simulink model "HyperscaleDataCenter"  (R2025b)
settings: Solver=VariableStepAuto  StartTime=0.0  StopTime=10  FixedStep=5e-5  RelTol=1e-4
PostLoadFcn:
  | HyperscaleDataCenterParam
values from neighbouring files (symbols this model uses):
  baseVoltageDC = 800    [DataCenterBBUParam.m]    (also in HyperscaleDataCenterParam.m; UPSBESSParam.m)
  bess_Ki = bess.controller.Ki    [SSTBESSParam.m]
  bess_Kp = bess.controller.Kp    [SSTBESSParam.m]
  droopGain = 0.02    [HyperscaleDataCenterParam.m]    (also in SSTBESSParam.m; UPSBESSParam.m)
  peakShavingPowerLimit = 800e3    (= 800000)    [HyperscaleDataCenterParam.m]
  powerTau = 0.005    [HyperscaleDataCenterParam.m]
  Prated_batt = 40e3    (= 40000)    [HyperscaleDataCenterParam.m]
  tauPS = 0.1    [HyperscaleDataCenterParam.m]
  Ts = 50e-6    (= 5e-05)    [BBUParam.m]    (also in DataCenterBBUParam.m; HyperscaleDataCenterParam.m)
  Ts_PS = 1e-3    (= 0.001)    [HyperscaleDataCenterParam.m]
undefined symbols (not defined in the file or in its folder): bbu, DiscIntNeverNeededParam, dspblkCoreblockFVToolHelper, ee_sli_rtmsupport, gcbh, grid, rack, sst, ups
libraries: fl_lib x80, nesl_utility x42, datacenter_lib x20, ee_lib x17, simulink x10, eeGeneralControl x9, slpidlib x6, microgridRenewables_lib x4, eeTransforms x4, batteryecm_lib x3, eeSinusoidalMeasurementV2 x2, simulink_extras x1
(part 3 of 5)

== system HyperscaleDataCenter/Server Load/Racks/Inference Rack ==
  U_in : Inport
  FaultFlag : Inport  Port=2
  Capacitor : fl_lib/Electrical/Electrical Elements/Capacitor  c=20e-3 F  r=1e-6 Ohm  g=0 1/Ohm  i_specify=off  i_priority=None  i=0 A  i_nominal_specify=off  i_nominal_value=1  i_nominal_unit=A  v_specify=off  v_priority=None  v=0 V  v_nominal_specify=off  v_nominal_value=1  v_nominal_unit=V  vc_specify=on  vc_priority=None  vc=800 V  vc_nominal_specify=off  vc_nominal_value=1  vc_nominal_unit=V
  Current Sensor : fl_lib/Electrical/Electrical Sensors/Current Sensor
  Dynamic Load : ee_lib/Passive/Dynamic Load  load_type=ee.enum.dc_ac.dc  min_supply_voltage=20 V  pow_min=1e-3 W  G_reverse=1e-6 S  deltaV=1e-3 V  f0=60 Hz  Vrms_min=200 V  tau=0.001 s  Vrms_ini=300 V  Vang_ini=0 deg
      settings: InternalSimscapePortConfiguration="{\"Bottom\":[],\"Left\":[{\"id\":\"p\",\"label\":\"+\",\"type\":\"foundation.electrical.electrical\"}],\"Right\":[{\"id\":\"n\",\"label\":\"-\",\"type\":\"foundation.electrical.electrical\"}],\"Top\":[{\"id\":\"P\",\"label\":\"P\",\"type\":\"input\"}]}"
  Efficiency Gain : fl_lib/Physical Signals/Functions/PS Gain  gain=rack.efficiencyGain
  Hybrid BBU : Subsystem  mask{includeSupercap=on, ctrl_Ts=Ts, ctrl_Vdc_ref=baseVoltageDC, scap_deadZone=bbu.scap.deadZone, scap_Kp=bbu.scap.Kp, scap_Imax=bbu.scap.Imax, scap_capacitance=bbu.scap.capacitance, scap_ESR=bbu.scap.ESR, scap_lpfAlpha=bbu.scap.lpfAlpha, batt_deadZone=bbu.batt.deadZone, batt_Imax=bbu.batt.Imax, batt_Vnom=bbu.batt.Vnom, batt_R1=bbu.batt.R1, batt_lpfAlpha=bbu.batt.lpfAlpha, batt_Kp_ctrl=bbu.batt.Kp_ctrl, batt_Ki_ctrl=bbu.batt.Ki_ctrl}
      mask prompts: includeSupercap "Include Supercapacitor"; ctrl_Ts "Controller sample time"; ctrl_Vdc_ref "DC bus voltage reference"; scap_deadZone "Dead Zone (V)"; scap_Kp "Droop Gain (A/V)"; scap_Imax "Current Limit (A)"; scap_capacitance "Capacitance (F)"; scap_ESR "ESR (Ohm)"; scap_lpfAlpha "SuperCap LPF alpha"; batt_deadZone "Dead Zone (V)"; batt_Imax "Current Limit (A)"; batt_Vnom "Nominal Voltage (V)"; batt_R1 "Internal Resistance (Ohm)"; batt_lpfAlpha "Battery LPF alpha"; batt_Kp_ctrl "Battery PI Kp"; batt_Ki_ctrl "Battery PI Ki"
      mask help: Hybrid Battery Backup Unit with frequency-separated supercapacitor (ms-range) and battery (sec-range) control.
      mask init:
      | % BBU Mask Initialization
      | 
      | % Handle supercapacitor inclusion
      | scPath = [gcb, '/Super Capacitor'];
      | if includeSupercap
      |     set_param(scPath, 'Commented', 'off');
      |     set_param([scPath, '/Droop Gate'], 'LowerValue', num2str(-scap_deadZone), 'UpperValue', num2str(scap_deadZone));
      |     set_param([scPath, '/Kp'], 'Gain', num2str(scap_Kp));
      |     set_param([scPath, '/Iref Sat'], 'UpperLimit', '0', 'LowerLimit', num2str(-scap_Imax));
      |     set_param([scPath, '/Capacitor'], 'c', num2str(scap_capacitance), 'r', num2str(scap_ESR));
      |     set_param([scPath, '/LPF'], 'Numerator', ['[' num2str(1-scap_lpfAlpha) ']'], 'Denominator', ['[1 ' num2str(-scap_lpfAlpha) ']']);
      | else
      |     set_param(scPath, 'Commented', 'on');
      | end
      | 
      | % Propagate battery parameters
      | btPath = [gcb, '/Battery'];
      | set_param([btPath, '/Droop Gate'], 'LowerValue', num2str(-batt_deadZone), 'UpperValue', num2str(batt_deadZone));
      | set_param([btPath, '/Iref Sat'], 'UpperLimit', '0', 'LowerLimit', num2str(-batt_Imax));
      | set_param([btPath, '/Battery'], 'Vnom', num2str(batt_Vnom), 'R1', num2str(batt_R1));
      | set_param([btPath, '/LPF'], 'Numerator', ['[' num2str(1-batt_lpfAlpha) ']'], 'Denominator', ['[1 ' num2str(-batt_lpfAlpha) ']']);
      mask Callback includeSupercap:
      | maskObj = Simulink.Mask.get(gcb);
      | scapEnabled = strcmp(get_param(gcb, 'includeSupercap'), 'on');
      | scapParams = {'scap_deadZone','scap_Kp','scap_Imax','scap_filterTau','scap_capacitance','scap_ESR'};
      | for i = 1:numel(scapParams)
      |     p = maskObj.getParameter(scapParams{i});
      |     if scapEnabled
      |         p.Visible = 'on';
      |     else
      |         p.Visible = 'off';
      |     end
      | end
      mask DialogControl ConfigTab Prompt: Configuration
      mask DialogControl SupercapTab Prompt: Supercapacitor
      mask DialogControl BatteryTab Prompt: Battery
      mask Display: image('hybrid_bbu_icon.png');
  PDU Racks : Subsystem  mask{nTrays=rack.nTrays, nRacks=rack.nRacks, trayMass=rack.trayMass, trayCp=rack.trayCp, trayThermalR=rack.trayThermalR, nGPU=rack.nGPU, gpuTDPperDie=rack.gpuTDPperDie, gpuIdlePower=rack.gpuIdlePower, gpuHBMpower=rack.gpuHBMpower, gpuExponent=rack.gpuExponent, gpuHBMutil=rack.gpuHBMutil, gpuLeakage=rack.gpuLeakage, gpuNominalDieT=rack.gpuNominalDieT, gpuDieThermalC=rack.gpuDieThermalC, gpuHeatSinkR=rack.gpuHeatSinkR, gpuSurfArea=rack.gpuSurfArea, gpuAmbientR=rack.gpuAmbientR, nCPU=rack.nCPU, cpuTDPperSocket=rack.cpuTDPperSocket, cpuIdlePower=rack.cpuIdlePower, cpuExponent=rack.cpuExponent, cpuLeakage=rack.cpuLeakage, cpuNominalDieT=rack.cpuNominalDieT, cpuDieThermalC=rack.cpuDieThermalC, cpuHeatSinkR=rack.cpuHeatSinkR, cpuSurfArea=rack.cpuSurfArea, cpuAmbientR=rack.cpuAmbientR, initialT=rack.initialT, htc=rack.htc}
      mask prompts: nTrays "Number of IT trays per rack (-)"; nRacks "Number of racks (-)"; trayMass "Tray mass (kg)"; trayCp "Tray specific heat capacity (J/kg*K)"; trayThermalR "Tray to external thermal resistance (K/W)"; nGPU "Number of GPU per tray (-)"; gpuTDPperDie "GPU TDP per die (W)"; gpuIdlePower "GPU idle power (W)"; gpuHBMpower "HBM power per GPU (W)"; gpuExponent "GPU power utilization exponent (-)"; gpuHBMutil "HBM utilization as fraction of compute utilization (-)"; gpuLeakage "Leakage increase per K above nominal temperature (W/K)"; gpuNominalDieT "Nominal die temperature at TDP (K)"; gpuDieThermalC "GPU die thermal capacitance (J/K)"; gpuHeatSinkR "GPU die-heat-sink thermal resistance (K/W)"; gpuSurfArea "Surface area per die for ambient heat transfer (m^2)"; gpuAmbientR "GPU die-ambient thermal resistance (K/W)"; nCPU "Number of CPU per tray (-)"; cpuTDPperSocket "CPU TDP per socket (W)"; cpuIdlePower "CPU idle power per socket (W)"; cpuExponent "CPU power utilization exponent (-)"; cpuLeakage "Leakage increase per K above nominal temperature (W/K)"; cpuNominalDieT "Nominal die temperature at TDP (K)"; cpuDieThermalC "CPU die thermal capacitance (J/K)"; cpuHeatSinkR "CPU die-heat-sink thermal resistance (K/W)"; cpuSurfArea "Surface area per die for ambient heat transfer (m^2)"; cpuAmbientR "CPU die-ambient thermal resistance (K/W)"; initialT "Initial temperature (K)"; htc "Heat transfer coefficient to ambient (W/m^2.K)"
      settings: CopyFcn=set_param(gcbh,'LinkStatus','none');  PortSchema="{\"entries\":[{\"content\":{\"sides\":[{\"content\":{\"connectorIds\":[\"LConn1\",\"LConn2\",\"LConn3\"]},\"type\":\"ConnectorPlacement.EquallySpacedRectSide\",\"uuid\":\"1a9a884a-dab1-4495-bf62-c6b2de6c1039\"},{\"content\":{\"connectorIds\":[\"RConn1\",\"RConn2\",\"RConn3\"],\"side\":\"RIGHT\"},\"type\":\"ConnectorPlacement.EquallySpacedRectSide\",\"uuid\":\"05c53434-51c1-4fee-b885-c321dcda8b6b\"},{\"content\":{\"side\":\"TOP\"},\"type\":\"ConnectorPlacement.EquallySpacedRectSide\",\"uuid\":\"c7b5c534-d596-4858-a133-27f005e6c9d4\"},{\"content\":{\"connectorIds\":[\"RConn4\"],\"side\":\"BOTTOM\"},\"type\":\"ConnectorPlacement.EquallySpacedRectSide\",\"uuid\":\"693f3c99-4296-4d86-bfcc-da753d3e576f\"}]},\"type\":\"ConnectorPlacement.EquallySpacedConnector\",\"uuid\":\"ed91c467-c4d0-403f-af16-bac0257594fd\"}],\"packageUris\":[\"http://schema.mathworks.com/mf0/Connector/R2020b\"],\"version\":\"1.0\"}"
      mask Help: web("DocumentationPDURacks.html")
      mask DialogControl Container10 Prompt: PDU Racks
      mask DialogControl getRatingButton Prompt: Get Rating
      mask DialogControl Container9 Prompt: IT Tray
      mask DialogControl Container6 Prompt: GPU
      mask DialogControl Container7 Prompt: CPU
      mask DialogControl Container8 Prompt: Initial Conditions
      mask Display: image('icon_PDURacks.png');
  PS-Simulink Converter1 : nesl_utility/PS-Simulink Converter  PhysicalDomain=network_engine_domain  SubClassName=ps_output  LeftPortType=input  RightPortType=output  PseudoPeriodic=off  Frequencies=[]  VectorFormat=inherit  Unit=inherit  AffineConversion=off
  PS-Simulink Converter2 : nesl_utility/PS-Simulink Converter  PhysicalDomain=network_engine_domain  SubClassName=ps_output  LeftPortType=input  RightPortType=output  PseudoPeriodic=off  Frequencies=[]  VectorFormat=inherit  Unit=inherit  AffineConversion=off
  Product : Product
  SP Conv U : nesl_utility/Simulink-PS Converter  PhysicalDomain=network_engine_domain  SubClassName=ps_input  LeftPortType=input  RightPortType=output  PseudoPeriodic=off  Frequencies=[]  NoiseDistribution=none  NoiseParameters=[]  Unit=1  AffineConversion=off  FilteringAndDerivatives=provide  SimscapeFilterOrder=1  InputFilterTimeConstant=0.001  UdotUserProvided=0
  TermC_Ha : fl_lib/Thermal/Thermal Elements/Thermal Mass  mass_type=foundation.enum.constant_variable.constant  mass=1e4 kg  sp_heat=1000 J/(K*kg)  mass_min=1e-6 kg  num_ports=foundation.enum.numPorts2.one  m_specify=off  m_priority=None  m=1 kg  m_nominal_specify=off  m_nominal_value=1  m_nominal_unit=kg  T_specify=off  T_priority=None  T=308.15 K  T_nominal_specify=off  T_nominal_value=1  T_nominal_unit=K  Q_specify=off  Q_priority=None  Q=0 W  Q_nominal_specify=off  Q_nominal_value=1  Q_nominal_unit=W
  TermC_Hc : fl_lib/Thermal/Thermal Elements/Thermal Mass  mass_type=foundation.enum.constant_variable.constant  mass=1e4 kg  sp_heat=1000 J/(K*kg)  mass_min=1e-6 kg  num_ports=foundation.enum.numPorts2.one  m_specify=off  m_priority=None  m=1 kg  m_nominal_specify=off  m_nominal_value=1  m_nominal_unit=kg  T_specify=off  T_priority=None  T=308.15 K  T_nominal_specify=off  T_nominal_value=1  T_nominal_unit=K  Q_specify=off  Q_priority=None  Q=0 W  Q_nominal_specify=off  Q_nominal_value=1  Q_nominal_unit=W
  Terminator : Terminator
  Voltage Sensor : fl_lib/Electrical/Electrical Sensors/Voltage Sensor
  + : PMIOPort  Side=Left
  - : PMIOPort  Port=2  Side=Left
  wires:
  PS-Simulink Converter2/1 -> Product/2, Hybrid BBU/1(Vdc_meas)  "Vdc_train"
  U_in/1 -> SP Conv U/1
  FaultFlag/1 -> Hybrid BBU/2(FaultFlag)
  PS-Simulink Converter1/1 -> Product/1
  Product/1 -> Terminator/1
  connections:
  PS-Simulink Converter2/LConn1 -- Voltage Sensor/RConn1
  Voltage Sensor/RConn2 -- Hybrid BBU/LConn2 -- Dynamic Load/RConn1 -- -/RConn1 -- Capacitor/RConn1
  SP Conv U/RConn1 -- PDU Racks/LConn2 -- PDU Racks/LConn1
  Capacitor/LConn1 -- Current Sensor/RConn2 -- Dynamic Load/LConn1
  PS-Simulink Converter1/LConn1 -- Current Sensor/RConn1
  Efficiency Gain/RConn1 -- Dynamic Load/LConn2
  Hybrid BBU/LConn1 -- +/RConn1 -- Current Sensor/LConn1 -- Voltage Sensor/LConn1
  PDU Racks/RConn1 -- Efficiency Gain/LConn1
  PDU Racks/LConn3 -- TermC_Ha/LConn1
  PDU Racks/RConn4 -- TermC_Hc/LConn1

== system HyperscaleDataCenter/Server Load/Racks/Training Rack ==
  U_in : Inport
  FaultFlag : Inport  Port=2
  Capacitor : fl_lib/Electrical/Electrical Elements/Capacitor  c=20e-3 F  r=1e-6 Ohm  g=0 1/Ohm  i_specify=off  i_priority=None  i=0 A  i_nominal_specify=off  i_nominal_value=1  i_nominal_unit=A  v_specify=off  v_priority=None  v=0 V  v_nominal_specify=off  v_nominal_value=1  v_nominal_unit=V  vc_specify=on  vc_priority=None  vc=800 V  vc_nominal_specify=off  vc_nominal_value=1  vc_nominal_unit=V
  Current Sensor : fl_lib/Electrical/Electrical Sensors/Current Sensor
  Dynamic Load : ee_lib/Passive/Dynamic Load  load_type=ee.enum.dc_ac.dc  min_supply_voltage=20 V  pow_min=1e-3 W  G_reverse=1e-6 S  deltaV=1e-3 V  f0=60 Hz  Vrms_min=200 V  tau=0.001 s  Vrms_ini=300 V  Vang_ini=0 deg
      settings: InternalSimscapePortConfiguration="{\"Bottom\":[],\"Left\":[{\"id\":\"p\",\"label\":\"+\",\"type\":\"foundation.electrical.electrical\"}],\"Right\":[{\"id\":\"n\",\"label\":\"-\",\"type\":\"foundation.electrical.electrical\"}],\"Top\":[{\"id\":\"P\",\"label\":\"P\",\"type\":\"input\"}]}"
  Efficiency Gain : fl_lib/Physical Signals/Functions/PS Gain  gain=rack.efficiencyGain
  Hybrid BBU : Subsystem  mask{includeSupercap=on, ctrl_Ts=Ts, ctrl_Vdc_ref=baseVoltageDC, scap_deadZone=bbu.scap.deadZone, scap_Kp=bbu.scap.Kp, scap_Imax=bbu.scap.Imax, scap_capacitance=bbu.scap.capacitance, scap_ESR=bbu.scap.ESR, scap_lpfAlpha=bbu.scap.lpfAlpha, batt_deadZone=bbu.batt.deadZone, batt_Imax=bbu.batt.Imax, batt_Vnom=bbu.batt.Vnom, batt_R1=bbu.batt.R1, batt_lpfAlpha=bbu.batt.lpfAlpha, batt_Kp_ctrl=bbu.batt.Kp_ctrl, batt_Ki_ctrl=bbu.batt.Ki_ctrl}
      mask prompts: includeSupercap "Include Supercapacitor"; ctrl_Ts "Controller sample time"; ctrl_Vdc_ref "DC bus voltage reference"; scap_deadZone "Dead Zone (V)"; scap_Kp "Droop Gain (A/V)"; scap_Imax "Current Limit (A)"; scap_capacitance "Capacitance (F)"; scap_ESR "ESR (Ohm)"; scap_lpfAlpha "SuperCap LPF alpha"; batt_deadZone "Dead Zone (V)"; batt_Imax "Current Limit (A)"; batt_Vnom "Nominal Voltage (V)"; batt_R1 "Internal Resistance (Ohm)"; batt_lpfAlpha "Battery LPF alpha"; batt_Kp_ctrl "Battery PI Kp"; batt_Ki_ctrl "Battery PI Ki"
      mask help: Hybrid Battery Backup Unit with frequency-separated supercapacitor (ms-range) and battery (sec-range) control.
      mask init: same as HyperscaleDataCenter/Server Load/Racks/Inference Rack/Hybrid BBU
      mask Callback includeSupercap:
      | maskObj = Simulink.Mask.get(gcb);
      | scapEnabled = strcmp(get_param(gcb, 'includeSupercap'), 'on');
      | scapParams = {'scap_deadZone','scap_Kp','scap_Imax','scap_filterTau','scap_capacitance','scap_ESR'};
      | for i = 1:numel(scapParams)
      |     p = maskObj.getParameter(scapParams{i});
      |     if scapEnabled
      |         p.Visible = 'on';
      |     else
      |         p.Visible = 'off';
      |     end
      | end
      mask DialogControl ConfigTab Prompt: Configuration
      mask DialogControl SupercapTab Prompt: Supercapacitor
      mask DialogControl BatteryTab Prompt: Battery
      mask Display: image('hybrid_bbu_icon.png');
  PDU Racks : Subsystem  mask{nTrays=rack.nTrays, nRacks=rack.nRacks, trayMass=rack.trayMass, trayCp=rack.trayCp, trayThermalR=rack.trayThermalR, nGPU=rack.nGPU, gpuTDPperDie=rack.gpuTDPperDie, gpuIdlePower=rack.gpuIdlePower, gpuHBMpower=rack.gpuHBMpower, gpuExponent=rack.gpuExponent, gpuHBMutil=rack.gpuHBMutil, gpuLeakage=rack.gpuLeakage, gpuNominalDieT=rack.gpuNominalDieT, gpuDieThermalC=rack.gpuDieThermalC, gpuHeatSinkR=rack.gpuHeatSinkR, gpuSurfArea=rack.gpuSurfArea, gpuAmbientR=rack.gpuAmbientR, nCPU=rack.nCPU, cpuTDPperSocket=rack.cpuTDPperSocket, cpuIdlePower=rack.cpuIdlePower, cpuExponent=rack.cpuExponent, cpuLeakage=rack.cpuLeakage, cpuNominalDieT=rack.cpuNominalDieT, cpuDieThermalC=rack.cpuDieThermalC, cpuHeatSinkR=rack.cpuHeatSinkR, cpuSurfArea=rack.cpuSurfArea, cpuAmbientR=rack.cpuAmbientR, initialT=rack.initialT, htc=rack.htc}
      mask prompts: nTrays "Number of IT trays per rack (-)"; nRacks "Number of racks (-)"; trayMass "Tray mass (kg)"; trayCp "Tray specific heat capacity (J/kg*K)"; trayThermalR "Tray to external thermal resistance (K/W)"; nGPU "Number of GPU per tray (-)"; gpuTDPperDie "GPU TDP per die (W)"; gpuIdlePower "GPU idle power (W)"; gpuHBMpower "HBM power per GPU (W)"; gpuExponent "GPU power utilization exponent (-)"; gpuHBMutil "HBM utilization as fraction of compute utilization (-)"; gpuLeakage "Leakage increase per K above nominal temperature (W/K)"; gpuNominalDieT "Nominal die temperature at TDP (K)"; gpuDieThermalC "GPU die thermal capacitance (J/K)"; gpuHeatSinkR "GPU die-heat-sink thermal resistance (K/W)"; gpuSurfArea "Surface area per die for ambient heat transfer (m^2)"; gpuAmbientR "GPU die-ambient thermal resistance (K/W)"; nCPU "Number of CPU per tray (-)"; cpuTDPperSocket "CPU TDP per socket (W)"; cpuIdlePower "CPU idle power per socket (W)"; cpuExponent "CPU power utilization exponent (-)"; cpuLeakage "Leakage increase per K above nominal temperature (W/K)"; cpuNominalDieT "Nominal die temperature at TDP (K)"; cpuDieThermalC "CPU die thermal capacitance (J/K)"; cpuHeatSinkR "CPU die-heat-sink thermal resistance (K/W)"; cpuSurfArea "Surface area per die for ambient heat transfer (m^2)"; cpuAmbientR "CPU die-ambient thermal resistance (K/W)"; initialT "Initial temperature (K)"; htc "Heat transfer coefficient to ambient (W/m^2.K)"
      settings: CopyFcn=set_param(gcbh,'LinkStatus','none');  PortSchema="{\"entries\":[{\"content\":{\"sides\":[{\"content\":{\"connectorIds\":[\"LConn1\",\"LConn2\",\"LConn3\"]},\"type\":\"ConnectorPlacement.EquallySpacedRectSide\",\"uuid\":\"1a9a884a-dab1-4495-bf62-c6b2de6c1039\"},{\"content\":{\"connectorIds\":[\"RConn1\",\"RConn2\",\"RConn3\"],\"side\":\"RIGHT\"},\"type\":\"ConnectorPlacement.EquallySpacedRectSide\",\"uuid\":\"05c53434-51c1-4fee-b885-c321dcda8b6b\"},{\"content\":{\"side\":\"TOP\"},\"type\":\"ConnectorPlacement.EquallySpacedRectSide\",\"uuid\":\"c7b5c534-d596-4858-a133-27f005e6c9d4\"},{\"content\":{\"connectorIds\":[\"RConn4\"],\"side\":\"BOTTOM\"},\"type\":\"ConnectorPlacement.EquallySpacedRectSide\",\"uuid\":\"693f3c99-4296-4d86-bfcc-da753d3e576f\"}]},\"type\":\"ConnectorPlacement.EquallySpacedConnector\",\"uuid\":\"ed91c467-c4d0-403f-af16-bac0257594fd\"}],\"packageUris\":[\"http://schema.mathworks.com/mf0/Connector/R2020b\"],\"version\":\"1.0\"}"
      mask Help: web("DocumentationPDURacks.html")
      mask DialogControl Container10 Prompt: PDU Racks
      mask DialogControl getRatingButton Prompt: Get Rating
      mask DialogControl Container9 Prompt: IT Tray
      mask DialogControl Container6 Prompt: GPU
      mask DialogControl Container7 Prompt: CPU
      mask DialogControl Container8 Prompt: Initial Conditions
      mask Display: image('icon_PDURacks.png');
  PS-Simulink Converter : nesl_utility/PS-Simulink Converter  PhysicalDomain=network_engine_domain  SubClassName=ps_output  LeftPortType=input  RightPortType=output  PseudoPeriodic=off  Frequencies=[]  VectorFormat=inherit  Unit=inherit  AffineConversion=off
  PS-Simulink Converter1 : nesl_utility/PS-Simulink Converter  PhysicalDomain=network_engine_domain  SubClassName=ps_output  LeftPortType=input  RightPortType=output  PseudoPeriodic=off  Frequencies=[]  VectorFormat=inherit  Unit=inherit  AffineConversion=off
  PS-Simulink Converter2 : nesl_utility/PS-Simulink Converter  PhysicalDomain=network_engine_domain  SubClassName=ps_output  LeftPortType=input  RightPortType=output  PseudoPeriodic=off  Frequencies=[]  VectorFormat=inherit  Unit=inherit  AffineConversion=off
  Product : Product
  SP Conv U : nesl_utility/Simulink-PS Converter  PhysicalDomain=network_engine_domain  SubClassName=ps_input  LeftPortType=input  RightPortType=output  PseudoPeriodic=off  Frequencies=[]  NoiseDistribution=none  NoiseParameters=[]  Unit=1  AffineConversion=off  FilteringAndDerivatives=provide  SimscapeFilterOrder=1  InputFilterTimeConstant=0.001  UdotUserProvided=0
  TermC_Ha : fl_lib/Thermal/Thermal Elements/Thermal Mass  mass_type=foundation.enum.constant_variable.constant  mass=1e4 kg  sp_heat=1000 J/(K*kg)  mass_min=1e-6 kg  num_ports=foundation.enum.numPorts2.one  m_specify=off  m_priority=None  m=1 kg  m_nominal_specify=off  m_nominal_value=1  m_nominal_unit=kg  T_specify=off  T_priority=None  T=308.15 K  T_nominal_specify=off  T_nominal_value=1  T_nominal_unit=K  Q_specify=off  Q_priority=None  Q=0 W  Q_nominal_specify=off  Q_nominal_value=1  Q_nominal_unit=W
  TermC_Hc : fl_lib/Thermal/Thermal Elements/Thermal Mass  mass_type=foundation.enum.constant_variable.constant  mass=1e4 kg  sp_heat=1000 J/(K*kg)  mass_min=1e-6 kg  num_ports=foundation.enum.numPorts2.one  m_specify=off  m_priority=None  m=1 kg  m_nominal_specify=off  m_nominal_value=1  m_nominal_unit=kg  T_specify=off  T_priority=None  T=308.15 K  T_nominal_specify=off  T_nominal_value=1  T_nominal_unit=K  Q_specify=off  Q_priority=None  Q=0 W  Q_nominal_specify=off  Q_nominal_value=1  Q_nominal_unit=W
  Terminator : Terminator
  Terminator1 : Terminator
  Voltage Sensor : fl_lib/Electrical/Electrical Sensors/Voltage Sensor
  + : PMIOPort  Side=Left
  - : PMIOPort  Port=2  Side=Left
  wires:
  U_in/1 -> SP Conv U/1
  FaultFlag/1 -> Hybrid BBU/2(FaultFlag)
  Product/1 -> Terminator/1
  PS-Simulink Converter/1 -> Terminator1/1
  PS-Simulink Converter1/1 -> Product/1
  PS-Simulink Converter2/1 -> Product/2, Hybrid BBU/1(Vdc_meas)
  connections:
  SP Conv U/RConn1 -- PDU Racks/LConn2 -- PDU Racks/LConn1
  -/RConn1 -- Voltage Sensor/RConn2 -- Hybrid BBU/LConn2 -- Capacitor/RConn1 -- Dynamic Load/RConn1
  Hybrid BBU/LConn1 -- Voltage Sensor/LConn1 -- Capacitor/LConn1 -- Dynamic Load/LConn1 -- Current Sensor/RConn2
  Efficiency Gain/RConn1 -- Dynamic Load/LConn2
  PS-Simulink Converter1/LConn1 -- Current Sensor/RConn1
  Voltage Sensor/RConn1 -- PS-Simulink Converter2/LConn1 -- PS-Simulink Converter/LConn1
  +/RConn1 -- Current Sensor/LConn1
  PDU Racks/RConn1 -- Efficiency Gain/LConn1
  PDU Racks/LConn3 -- TermC_Ha/LConn1
  PDU Racks/RConn4 -- TermC_Hc/LConn1

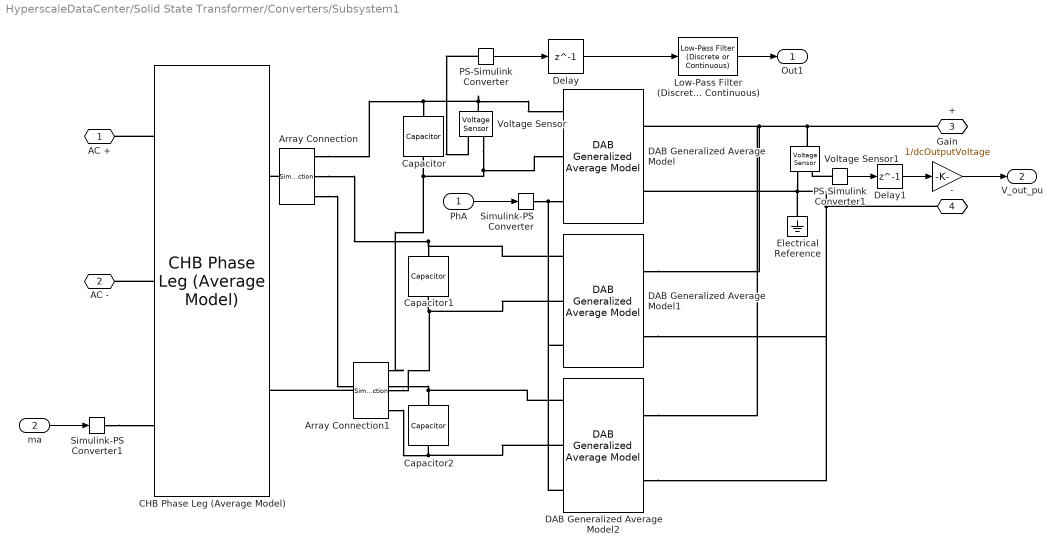
== system HyperscaleDataCenter/Solid State Transformer/Converters/Subsystem1 ==
  PhA : Inport
  ma : Inport  Port=2
  Array Connection : SimscapeArrayConnection  NumScalarElements=3
  Array Connection1 : SimscapeArrayConnection  NumScalarElements=3
  CHB Phase Leg (Average Model) : datacenter_lib/CHB Phase Leg (Average Model)  NumModules=3  OnResistance=1e-3 Ohm  InitialDCVoltage=4400 V  GridVoltage=13800 V  TotalDCVoltage=13200 V
      settings: InternalSimscapePortConfiguration="{\"Bottom\":[],\"Left\":[{\"id\":\"ACPositive\",\"label\":\"AC+\",\"type\":\"foundation.electrical.electrical\"},{\"id\":\"ACNegative\",\"label\":\"AC-\",\"type\":\"foundation.electrical.electrical\"},{\"id\":\"m\",\"label\":\"m\",\"type\":\"input\"}],\"Right\":[{\"id\":\"DCPositive\",\"label\":\"DC+\",\"type\":\"foundation.electrical.electrical\"},{\"id\":\"DCNegative\",\"label\":\"DC-\",\"type\":\"foundation.electrical.electrical\"}],\"Top\":[]}"
  Capacitor : fl_lib/Electrical/Electrical Elements/Capacitor  c=0.005 F  r=1e-6 Ohm  g=0 1/Ohm  i_specify=off  i_priority=None  i=0 A  i_nominal_specify=off  i_nominal_value=1  i_nominal_unit=A  v_specify=off  v_priority=None  v=0 V  v_nominal_specify=off  v_nominal_value=1  v_nominal_unit=V  vc_specify=on  vc_priority=None  vc=4400 V  vc_nominal_specify=off  vc_nominal_value=1  vc_nominal_unit=V
  Capacitor1 : fl_lib/Electrical/Electrical Elements/Capacitor  c=0.005 F  r=1e-6 Ohm  g=0 1/Ohm  i_specify=off  i_priority=None  i=0 A  i_nominal_specify=off  i_nominal_value=1  i_nominal_unit=A  v_specify=off  v_priority=None  v=0 V  v_nominal_specify=off  v_nominal_value=1  v_nominal_unit=V  vc_specify=on  vc_priority=None  vc=4400 V  vc_nominal_specify=off  vc_nominal_value=1  vc_nominal_unit=V
  Capacitor2 : fl_lib/Electrical/Electrical Elements/Capacitor  c=0.005 F  r=1e-6 Ohm  g=0 1/Ohm  i_specify=off  i_priority=None  i=0 A  i_nominal_specify=off  i_nominal_value=1  i_nominal_unit=A  v_specify=off  v_priority=None  v=0 V  v_nominal_specify=off  v_nominal_value=1  v_nominal_unit=V  vc_specify=on  vc_priority=None  vc=4400 V  vc_nominal_specify=off  vc_nominal_value=1  vc_nominal_unit=V
  DAB Generalized Average Model : datacenter_lib/DAB Generalized Average Model  N=sst.dab.turnsRatio  L1=sst.dab.primaryLeakageInductance H  L2=sst.dab.secondaryLeakageInductance H  Rt=sst.dab.windingResistance Ohm  Co=sst.dab.outputCapacitance F  fs=sst.dab.switchingFrequency Hz  vo0_init=sst.dab.vo0_init V  it1R_init=sst.dab.it1R_init A  it1I_init=sst.dab.it1I_init A  include_esr=false  Rc=0.25 Ohm  i_in_specify=on  i_in_priority=None  i_in=0 A  i_in_nominal_specify=off  i_in_nominal_value=1  i_in_nominal_unit=A  i_out_specify=on  i_out_priority=None  i_out=0 A  i_out_nominal_specify=off  i_out_nominal_value=1  i_out_nominal_unit=A  v_in_specify=on  v_in_priority=None  v_in=0 V  v_in_nominal_specify=off  v_in_nominal_value=1  v_in_nominal_unit=V  v_out_specify=on  v_out_priority=None  v_out=0 V  v_out_nominal_specify=off  v_out_nominal_value=1  v_out_nominal_unit=V
      settings: InternalSimscapePortConfiguration="{\"Bottom\":[],\"Left\":[{\"id\":\"p_in\",\"label\":\"V+\",\"type\":\"foundation.electrical.electrical\"},{\"id\":\"n_in\",\"label\":\"V-\",\"type\":\"foundation.electrical.electrical\"},{\"id\":\"d\",\"label\":\"d\",\"type\":\"input\"}],\"Right\":[{\"id\":\"p_out\",\"label\":\"Vo+\",\"type\":\"foundation.electrical.electrical\"},{\"id\":\"n_out\",\"label\":\"Vo-\",\"type\":\"foundation.electrical.electrical\"}],\"Top\":[]}"
  DAB Generalized Average Model1 : datacenter_lib/DAB Generalized Average Model  N=sst.dab.turnsRatio  L1=sst.dab.primaryLeakageInductance H  L2=sst.dab.secondaryLeakageInductance H  Rt=sst.dab.windingResistance Ohm  Co=sst.dab.outputCapacitance F  fs=sst.dab.switchingFrequency Hz  vo0_init=sst.dab.vo0_init V  it1R_init=sst.dab.it1R_init A  it1I_init=sst.dab.it1I_init A  include_esr=false  Rc=0.25 Ohm  i_in_specify=on  i_in_priority=None  i_in=0 A  i_in_nominal_specify=off  i_in_nominal_value=1  i_in_nominal_unit=A  i_out_specify=on  i_out_priority=None  i_out=0 A  i_out_nominal_specify=off  i_out_nominal_value=1  i_out_nominal_unit=A  v_in_specify=on  v_in_priority=None  v_in=0 V  v_in_nominal_specify=off  v_in_nominal_value=1  v_in_nominal_unit=V  v_out_specify=on  v_out_priority=None  v_out=0 V  v_out_nominal_specify=off  v_out_nominal_value=1  v_out_nominal_unit=V
      settings: InternalSimscapePortConfiguration="{\"Bottom\":[],\"Left\":[{\"id\":\"p_in\",\"label\":\"V+\",\"type\":\"foundation.electrical.electrical\"},{\"id\":\"n_in\",\"label\":\"V-\",\"type\":\"foundation.electrical.electrical\"},{\"id\":\"d\",\"label\":\"d\",\"type\":\"input\"}],\"Right\":[{\"id\":\"p_out\",\"label\":\"Vo+\",\"type\":\"foundation.electrical.electrical\"},{\"id\":\"n_out\",\"label\":\"Vo-\",\"type\":\"foundation.electrical.electrical\"}],\"Top\":[]}"
  DAB Generalized Average Model2 : datacenter_lib/DAB Generalized Average Model  N=sst.dab.turnsRatio  L1=sst.dab.primaryLeakageInductance H  L2=sst.dab.secondaryLeakageInductance H  Rt=sst.dab.windingResistance Ohm  Co=sst.dab.outputCapacitance F  fs=sst.dab.switchingFrequency Hz  vo0_init=sst.dab.vo0_init V  it1R_init=sst.dab.it1R_init A  it1I_init=sst.dab.it1I_init A  include_esr=false  Rc=0.25 Ohm  i_in_specify=on  i_in_priority=None  i_in=0 A  i_in_nominal_specify=off  i_in_nominal_value=1  i_in_nominal_unit=A  i_out_specify=on  i_out_priority=None  i_out=0 A  i_out_nominal_specify=off  i_out_nominal_value=1  i_out_nominal_unit=A  v_in_specify=on  v_in_priority=None  v_in=0 V  v_in_nominal_specify=off  v_in_nominal_value=1  v_in_nominal_unit=V  v_out_specify=on  v_out_priority=None  v_out=0 V  v_out_nominal_specify=off  v_out_nominal_value=1  v_out_nominal_unit=V
      settings: InternalSimscapePortConfiguration="{\"Bottom\":[],\"Left\":[{\"id\":\"p_in\",\"label\":\"V+\",\"type\":\"foundation.electrical.electrical\"},{\"id\":\"n_in\",\"label\":\"V-\",\"type\":\"foundation.electrical.electrical\"},{\"id\":\"d\",\"label\":\"d\",\"type\":\"input\"}],\"Right\":[{\"id\":\"p_out\",\"label\":\"Vo+\",\"type\":\"foundation.electrical.electrical\"},{\"id\":\"n_out\",\"label\":\"Vo-\",\"type\":\"foundation.electrical.electrical\"}],\"Top\":[]}"
  Delay : Delay  DelayLength=1
  Delay1 : Delay  DelayLength=1  InitialCondition=1
  Electrical Reference : fl_lib/Electrical/Electrical Elements/Electrical Reference
  Gain : Gain  Gain=1/dcOutputVoltage
  Low-Pass Filter (Discrete or Continuous) : eeGeneralControl/Low-Pass Filter (Discrete or Continuous)  K=1  T=0.005  B=inf  A=-inf  init_option=Inherited from block input  x0=0  Ts=-1
  PS-Simulink Converter : nesl_utility/PS-Simulink Converter  PhysicalDomain=network_engine_domain  SubClassName=ps_output  LeftPortType=input  RightPortType=output  PseudoPeriodic=off  Frequencies=[]  VectorFormat=inherit  Unit=inherit  AffineConversion=off
  PS-Simulink Converter1 : nesl_utility/PS-Simulink Converter  PhysicalDomain=network_engine_domain  SubClassName=ps_output  LeftPortType=input  RightPortType=output  PseudoPeriodic=off  Frequencies=[]  VectorFormat=inherit  Unit=inherit  AffineConversion=off
  Simulink-PS Converter : nesl_utility/Simulink-PS Converter  PhysicalDomain=network_engine_domain  SubClassName=ps_input  LeftPortType=input  RightPortType=output  PseudoPeriodic=off  Frequencies=[]  NoiseDistribution=none  NoiseParameters=[]  Unit=1  AffineConversion=off  FilteringAndDerivatives=provide  SimscapeFilterOrder=1  InputFilterTimeConstant=0.001  UdotUserProvided=0
  Simulink-PS Converter1 : nesl_utility/Simulink-PS Converter  PhysicalDomain=network_engine_domain  SubClassName=ps_input  LeftPortType=input  RightPortType=output  PseudoPeriodic=off  Frequencies=[]  NoiseDistribution=none  NoiseParameters=[]  Unit=1  AffineConversion=off  FilteringAndDerivatives=provide  SimscapeFilterOrder=1  InputFilterTimeConstant=0.001  UdotUserProvided=0
  Voltage Sensor : fl_lib/Electrical/Electrical Sensors/Voltage Sensor
  Voltage Sensor1 : fl_lib/Electrical/Electrical Sensors/Voltage Sensor
  AC + : PMIOPort  Side=Left
  AC - : PMIOPort  Port=2  Side=Left
  + : PMIOPort  Port=3  Side=Right
  - : PMIOPort  Port=4  Side=Right
  Out1 : Outport
  V_out_pu : Outport  Port=2
  wires:
  PS-Simulink Converter/1 -> Delay/1
  Delay/1 -> Low-Pass Filter (Discrete or Continuous)/1
  Low-Pass Filter (Discrete or Continuous)/1 -> Out1/1
  PS-Simulink Converter1/1 -> Delay1/1
  Delay1/1 -> Gain/1
  PhA/1 -> Simulink-PS Converter/1
  Gain/1 -> V_out_pu/1
  ma/1 -> Simulink-PS Converter1/1
  connections:
  PS-Simulink Converter/LConn1 -- Voltage Sensor/RConn1
  DAB Generalized Average Model1/LConn1 -- Array Connection/LConn2 -- Capacitor1/LConn1
  DAB Generalized Average Model1/LConn2 -- Array Connection1/LConn2 -- Capacitor1/RConn1
  Voltage Sensor/LConn1 -- Array Connection/LConn1 -- Capacitor/LConn1 -- DAB Generalized Average Model/LConn1
  CHB Phase Leg (Average Model)/LConn1 -- AC +/RConn1
  DAB Generalized Average Model2/LConn2 -- Array Connection1/LConn3 -- Capacitor2/RConn1
  DAB Generalized Average Model2/LConn1 -- Array Connection/LConn3 -- Capacitor2/LConn1
  CHB Phase Leg (Average Model)/LConn2 -- AC -/RConn1
  Voltage Sensor/RConn2 -- Capacitor/RConn1 -- Array Connection1/LConn1 -- DAB Generalized Average Model/LConn2
  +/RConn1 -- Voltage Sensor1/LConn1 -- DAB Generalized Average Model2/RConn1 -- DAB Generalized Average Model1/RConn1 -- DAB Generalized Average Model/RConn1
  -/RConn1 -- Electrical Reference/LConn1 -- Voltage Sensor1/RConn2 -- DAB Generalized Average Model/RConn2 -- DAB Generalized Average Model2/RConn2 -- DAB Generalized Average Model1/RConn2
  PS-Simulink Converter1/LConn1 -- Voltage Sensor1/RConn1
  Simulink-PS Converter/RConn1 -- DAB Generalized Average Model2/LConn3 -- DAB Generalized Average Model1/LConn3 -- DAB Generalized Average Model/LConn3
  Array Connection/RConn1 -- CHB Phase Leg (Average Model)/RConn1
  Array Connection1/RConn1 -- CHB Phase Leg (Average Model)/RConn2
  Simulink-PS Converter1/RConn1 -- CHB Phase Leg (Average Model)/LConn3

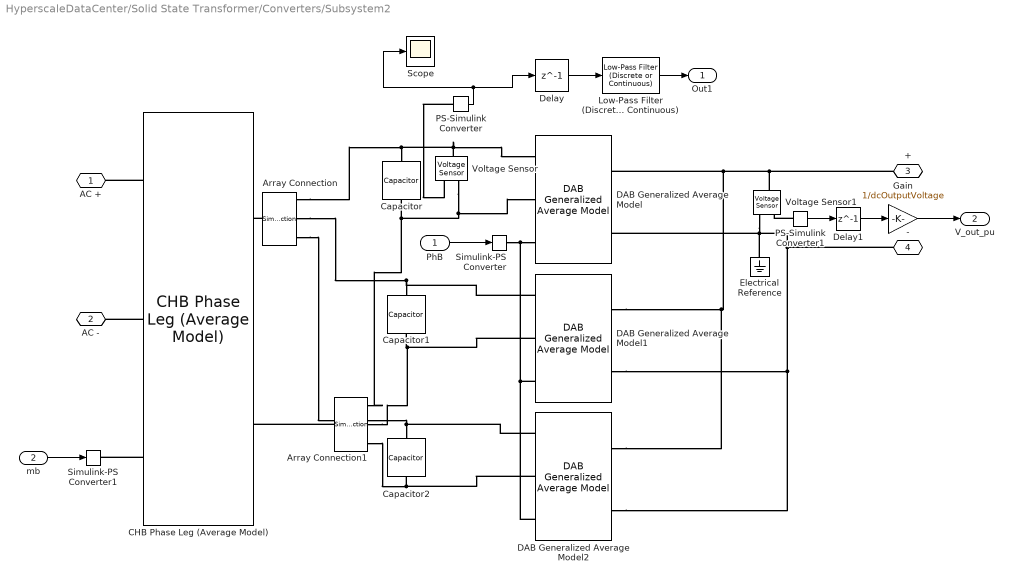
== system HyperscaleDataCenter/Solid State Transformer/Converters/Subsystem2 ==
  PhB : Inport
  mb : Inport  Port=2
  Array Connection : SimscapeArrayConnection  NumScalarElements=3
  Array Connection1 : SimscapeArrayConnection  NumScalarElements=3
  CHB Phase Leg (Average Model) : datacenter_lib/CHB Phase Leg (Average Model)  NumModules=3  OnResistance=1e-3 Ohm  InitialDCVoltage=4400 V  GridVoltage=13800 V  TotalDCVoltage=13200 V
      settings: InternalSimscapePortConfiguration="{\"Bottom\":[],\"Left\":[{\"id\":\"ACPositive\",\"label\":\"AC+\",\"type\":\"foundation.electrical.electrical\"},{\"id\":\"ACNegative\",\"label\":\"AC-\",\"type\":\"foundation.electrical.electrical\"},{\"id\":\"m\",\"label\":\"m\",\"type\":\"input\"}],\"Right\":[{\"id\":\"DCPositive\",\"label\":\"DC+\",\"type\":\"foundation.electrical.electrical\"},{\"id\":\"DCNegative\",\"label\":\"DC-\",\"type\":\"foundation.electrical.electrical\"}],\"Top\":[]}"
  Capacitor : fl_lib/Electrical/Electrical Elements/Capacitor  c=0.005 F  r=1e-6 Ohm  g=0 1/Ohm  i_specify=off  i_priority=None  i=0 A  i_nominal_specify=off  i_nominal_value=1  i_nominal_unit=A  v_specify=off  v_priority=None  v=0 V  v_nominal_specify=off  v_nominal_value=1  v_nominal_unit=V  vc_specify=on  vc_priority=None  vc=4400 V  vc_nominal_specify=off  vc_nominal_value=1  vc_nominal_unit=V
  Capacitor1 : fl_lib/Electrical/Electrical Elements/Capacitor  c=0.005 F  r=1e-6 Ohm  g=0 1/Ohm  i_specify=off  i_priority=None  i=0 A  i_nominal_specify=off  i_nominal_value=1  i_nominal_unit=A  v_specify=off  v_priority=None  v=0 V  v_nominal_specify=off  v_nominal_value=1  v_nominal_unit=V  vc_specify=on  vc_priority=None  vc=4400 V  vc_nominal_specify=off  vc_nominal_value=1  vc_nominal_unit=V
  Capacitor2 : fl_lib/Electrical/Electrical Elements/Capacitor  c=0.005 F  r=1e-6 Ohm  g=0 1/Ohm  i_specify=off  i_priority=None  i=0 A  i_nominal_specify=off  i_nominal_value=1  i_nominal_unit=A  v_specify=off  v_priority=None  v=0 V  v_nominal_specify=off  v_nominal_value=1  v_nominal_unit=V  vc_specify=on  vc_priority=None  vc=4400 V  vc_nominal_specify=off  vc_nominal_value=1  vc_nominal_unit=V
  DAB Generalized Average Model : datacenter_lib/DAB Generalized Average Model  N=sst.dab.turnsRatio  L1=sst.dab.primaryLeakageInductance H  L2=sst.dab.secondaryLeakageInductance H  Rt=sst.dab.windingResistance Ohm  Co=sst.dab.outputCapacitance F  fs=sst.dab.switchingFrequency Hz  vo0_init=sst.dab.vo0_init V  it1R_init=sst.dab.it1R_init A  it1I_init=sst.dab.it1I_init A  include_esr=false  Rc=0.25 Ohm  i_in_specify=on  i_in_priority=None  i_in=0 A  i_in_nominal_specify=off  i_in_nominal_value=1  i_in_nominal_unit=A  i_out_specify=on  i_out_priority=None  i_out=0 A  i_out_nominal_specify=off  i_out_nominal_value=1  i_out_nominal_unit=A  v_in_specify=on  v_in_priority=None  v_in=0 V  v_in_nominal_specify=off  v_in_nominal_value=1  v_in_nominal_unit=V  v_out_specify=on  v_out_priority=None  v_out=0 V  v_out_nominal_specify=off  v_out_nominal_value=1  v_out_nominal_unit=V
      settings: InternalSimscapePortConfiguration="{\"Bottom\":[],\"Left\":[{\"id\":\"p_in\",\"label\":\"V+\",\"type\":\"foundation.electrical.electrical\"},{\"id\":\"n_in\",\"label\":\"V-\",\"type\":\"foundation.electrical.electrical\"},{\"id\":\"d\",\"label\":\"d\",\"type\":\"input\"}],\"Right\":[{\"id\":\"p_out\",\"label\":\"Vo+\",\"type\":\"foundation.electrical.electrical\"},{\"id\":\"n_out\",\"label\":\"Vo-\",\"type\":\"foundation.electrical.electrical\"}],\"Top\":[]}"
  DAB Generalized Average Model1 : datacenter_lib/DAB Generalized Average Model  N=sst.dab.turnsRatio  L1=sst.dab.primaryLeakageInductance H  L2=sst.dab.secondaryLeakageInductance H  Rt=sst.dab.windingResistance Ohm  Co=sst.dab.outputCapacitance F  fs=sst.dab.switchingFrequency Hz  vo0_init=sst.dab.vo0_init V  it1R_init=sst.dab.it1R_init A  it1I_init=sst.dab.it1I_init A  include_esr=false  Rc=0.25 Ohm  i_in_specify=on  i_in_priority=None  i_in=0 A  i_in_nominal_specify=off  i_in_nominal_value=1  i_in_nominal_unit=A  i_out_specify=on  i_out_priority=None  i_out=0 A  i_out_nominal_specify=off  i_out_nominal_value=1  i_out_nominal_unit=A  v_in_specify=on  v_in_priority=None  v_in=0 V  v_in_nominal_specify=off  v_in_nominal_value=1  v_in_nominal_unit=V  v_out_specify=on  v_out_priority=None  v_out=0 V  v_out_nominal_specify=off  v_out_nominal_value=1  v_out_nominal_unit=V
      settings: InternalSimscapePortConfiguration="{\"Bottom\":[],\"Left\":[{\"id\":\"p_in\",\"label\":\"V+\",\"type\":\"foundation.electrical.electrical\"},{\"id\":\"n_in\",\"label\":\"V-\",\"type\":\"foundation.electrical.electrical\"},{\"id\":\"d\",\"label\":\"d\",\"type\":\"input\"}],\"Right\":[{\"id\":\"p_out\",\"label\":\"Vo+\",\"type\":\"foundation.electrical.electrical\"},{\"id\":\"n_out\",\"label\":\"Vo-\",\"type\":\"foundation.electrical.electrical\"}],\"Top\":[]}"
  DAB Generalized Average Model2 : datacenter_lib/DAB Generalized Average Model  N=sst.dab.turnsRatio  L1=sst.dab.primaryLeakageInductance H  L2=sst.dab.secondaryLeakageInductance H  Rt=sst.dab.windingResistance Ohm  Co=sst.dab.outputCapacitance F  fs=sst.dab.switchingFrequency Hz  vo0_init=sst.dab.vo0_init V  it1R_init=sst.dab.it1R_init A  it1I_init=sst.dab.it1I_init A  include_esr=false  Rc=0.25 Ohm  i_in_specify=on  i_in_priority=None  i_in=0 A  i_in_nominal_specify=off  i_in_nominal_value=1  i_in_nominal_unit=A  i_out_specify=on  i_out_priority=None  i_out=0 A  i_out_nominal_specify=off  i_out_nominal_value=1  i_out_nominal_unit=A  v_in_specify=on  v_in_priority=None  v_in=0 V  v_in_nominal_specify=off  v_in_nominal_value=1  v_in_nominal_unit=V  v_out_specify=on  v_out_priority=None  v_out=0 V  v_out_nominal_specify=off  v_out_nominal_value=1  v_out_nominal_unit=V
      settings: InternalSimscapePortConfiguration="{\"Bottom\":[],\"Left\":[{\"id\":\"p_in\",\"label\":\"V+\",\"type\":\"foundation.electrical.electrical\"},{\"id\":\"n_in\",\"label\":\"V-\",\"type\":\"foundation.electrical.electrical\"},{\"id\":\"d\",\"label\":\"d\",\"type\":\"input\"}],\"Right\":[{\"id\":\"p_out\",\"label\":\"Vo+\",\"type\":\"foundation.electrical.electrical\"},{\"id\":\"n_out\",\"label\":\"Vo-\",\"type\":\"foundation.electrical.electrical\"}],\"Top\":[]}"
  Delay : Delay  DelayLength=1
  Delay1 : Delay  DelayLength=1  InitialCondition=1
  Electrical Reference : fl_lib/Electrical/Electrical Elements/Electrical Reference
  Gain : Gain  Gain=1/dcOutputVoltage
  Low-Pass Filter (Discrete or Continuous) : eeGeneralControl/Low-Pass Filter (Discrete or Continuous)  K=1  T=0.005  B=inf  A=-inf  init_option=Inherited from block input  x0=0  Ts=-1
  PS-Simulink Converter : nesl_utility/PS-Simulink Converter  PhysicalDomain=network_engine_domain  SubClassName=ps_output  LeftPortType=input  RightPortType=output  PseudoPeriodic=off  Frequencies=[]  VectorFormat=inherit  Unit=inherit  AffineConversion=off
  PS-Simulink Converter1 : nesl_utility/PS-Simulink Converter  PhysicalDomain=network_engine_domain  SubClassName=ps_output  LeftPortType=input  RightPortType=output  PseudoPeriodic=off  Frequencies=[]  VectorFormat=inherit  Unit=inherit  AffineConversion=off
  Scope : Scope
      settings: ActiveDisplayYMinimum=-1  ActiveDisplayYMaximum=1
  Simulink-PS Converter : nesl_utility/Simulink-PS Converter  PhysicalDomain=network_engine_domain  SubClassName=ps_input  LeftPortType=input  RightPortType=output  PseudoPeriodic=off  Frequencies=[]  NoiseDistribution=none  NoiseParameters=[]  Unit=1  AffineConversion=off  FilteringAndDerivatives=provide  SimscapeFilterOrder=1  InputFilterTimeConstant=0.001  UdotUserProvided=0
  Simulink-PS Converter1 : nesl_utility/Simulink-PS Converter  PhysicalDomain=network_engine_domain  SubClassName=ps_input  LeftPortType=input  RightPortType=output  PseudoPeriodic=off  Frequencies=[]  NoiseDistribution=none  NoiseParameters=[]  Unit=1  AffineConversion=off  FilteringAndDerivatives=provide  SimscapeFilterOrder=1  InputFilterTimeConstant=0.001  UdotUserProvided=0
  Voltage Sensor : fl_lib/Electrical/Electrical Sensors/Voltage Sensor
  Voltage Sensor1 : fl_lib/Electrical/Electrical Sensors/Voltage Sensor
  AC + : PMIOPort  Side=Left
  AC - : PMIOPort  Port=2  Side=Left
  + : PMIOPort  Port=3  Side=Right
  - : PMIOPort  Port=4  Side=Right
  Out1 : Outport
  V_out_pu : Outport  Port=2
  wires:
  PS-Simulink Converter/1 -> Delay/1, Scope/1
  Delay/1 -> Low-Pass Filter (Discrete or Continuous)/1
  Low-Pass Filter (Discrete or Continuous)/1 -> Out1/1
  PS-Simulink Converter1/1 -> Delay1/1
  Delay1/1 -> Gain/1
  PhB/1 -> Simulink-PS Converter/1
  Gain/1 -> V_out_pu/1
  mb/1 -> Simulink-PS Converter1/1
  connections:
  PS-Simulink Converter/LConn1 -- Voltage Sensor/RConn1
  DAB Generalized Average Model1/LConn1 -- Capacitor1/LConn1 -- Array Connection/LConn2
  Capacitor1/RConn1 -- DAB Generalized Average Model1/LConn2 -- Array Connection1/LConn2
  Capacitor/LConn1 -- Voltage Sensor/LConn1 -- DAB Generalized Average Model/LConn1 -- Array Connection/LConn1
  CHB Phase Leg (Average Model)/LConn1 -- AC +/RConn1
  DAB Generalized Average Model2/LConn2 -- Capacitor2/RConn1 -- Array Connection1/LConn3
  Capacitor2/LConn1 -- DAB Generalized Average Model2/LConn1 -- Array Connection/LConn3
  CHB Phase Leg (Average Model)/LConn2 -- AC -/RConn1
  Array Connection1/LConn1 -- Voltage Sensor/RConn2 -- DAB Generalized Average Model/LConn2 -- Capacitor/RConn1
  +/RConn1 -- Voltage Sensor1/LConn1 -- DAB Generalized Average Model2/RConn1 -- DAB Generalized Average Model1/RConn1 -- DAB Generalized Average Model/RConn1
  -/RConn1 -- Electrical Reference/LConn1 -- Voltage Sensor1/RConn2 -- DAB Generalized Average Model/RConn2 -- DAB Generalized Average Model2/RConn2 -- DAB Generalized Average Model1/RConn2
  PS-Simulink Converter1/LConn1 -- Voltage Sensor1/RConn1
  Simulink-PS Converter/RConn1 -- DAB Generalized Average Model2/LConn3 -- DAB Generalized Average Model1/LConn3 -- DAB Generalized Average Model/LConn3
  Array Connection/RConn1 -- CHB Phase Leg (Average Model)/RConn1
  Array Connection1/RConn1 -- CHB Phase Leg (Average Model)/RConn2
  CHB Phase Leg (Average Model)/LConn3 -- Simulink-PS Converter1/RConn1
